simulink model "RTInductionMotorJan27"  (R2020a)
settings: Solver=FixedStepAuto  StartTime=0.0  StopTime=1  RelTol=1e-3
model workspace (MAT data in the model file):
  Fe = 60
  Poles = 2
libraries: powerlib x26, powerlib_meascontrol x4, simulink x1
(part 2 of 2)

== system RTInductionMotorJan27/Motor Model/first test (g results with simscape but without feedback)/Rotor current/Rotor currents ==
  flux_dr : Inport
  flus_qr : Inport  Port=2
  Lr : Inport  Port=3
  Lm : Inport  Port=4
  Add : Sum
  Divide : Product  Inputs=*/
  Divide1 : Product  Inputs=/*
  Lm1 : InportShadow  Port=4
  Product : Product
  Product1 : Product
  Scope : Scope  NumInputPorts=2
  Subtract : Sum  Inputs=-+
  Subtract1 : Sum  Inputs=-+
  i_dr : Outport  VectorParamsAs1DForOutWhenUnconnected=off
  i_qr : Outport  Port=2  VectorParamsAs1DForOutWhenUnconnected=off
  tag scope: i_dr=global, i_qr=global
  wires:
  Divide1/1 -> i_qr/1, Scope/1, [i_qr]  "i_rs"
  Subtract1/1 -> Divide1/2
  flus_qr/1 -> Subtract1/2
  Product1/1 -> Subtract1/1
  [i_qs] -> Product1/2
  Divide/1 -> i_dr/1, Scope/2, [i_dr]  "i_dr"
  Add/1 -> Divide/2, Divide1/1
  Subtract/1 -> Divide/1
  Lm/1 -> Add/2, Product1/1
  Lr/1 -> Add/1
  Product/1 -> Subtract/1
  flux_dr/1 -> Subtract/2
  [i_ds] -> Product/2
  Lm1/1 -> Product/1

== system RTInductionMotorJan27/Motor Model/first test (g results with simscape but without feedback)/Stator current/Stator Flux ==
  Rs (Ohms) : Inport
  w_s : Inport  Port=2
  dq0 : Inport  Port=3
  Demux : Demux  Outputs=3
  Integrator : Integrator
  Integrator1 : Integrator
  Rs (Ohms)1 : InportShadow
  Scope : Scope  NumInputPorts=2
  Subtract : Sum  Inputs=-++
  Subtract1 : Sum  Inputs=-+-
  Terminator : Terminator
  product{,1..3} (4 alike) : Product  Inputs=**
  w_s1 : InportShadow  Port=2
  flux_ds : Outport  VectorParamsAs1DForOutWhenUnconnected=off
  flux_qs : Outport  Port=2  VectorParamsAs1DForOutWhenUnconnected=off
  wires:
  Demux/3 -> Terminator/1
  Demux/2 -> Subtract1/2  "v_qs"
  Demux/1 -> Subtract/2  "v_ds"
  [i_qs] -> product1/2
  product2/1 -> Subtract1/1
  w_s/1 -> product2/2
  product3/1 -> Subtract/3
  w_s1/1 -> product3/1
  Rs (Ohms)1/1 -> product1/1
  Integrator1/1 -> flux_qs/1, Scope/2, product3/2  "flux_qs"
  [i_ds] -> product/1
  product1/1 -> Subtract1/3
  Subtract1/1 -> Integrator1/1
  Integrator/1 -> flux_ds/1, Scope/1, product2/1  "flux_ds"
  Subtract/1 -> Integrator/1
  product/1 -> Subtract/1  "i_ds*R_s"
  Rs (Ohms)/1 -> product/2
  dq0/1 -> Demux/1

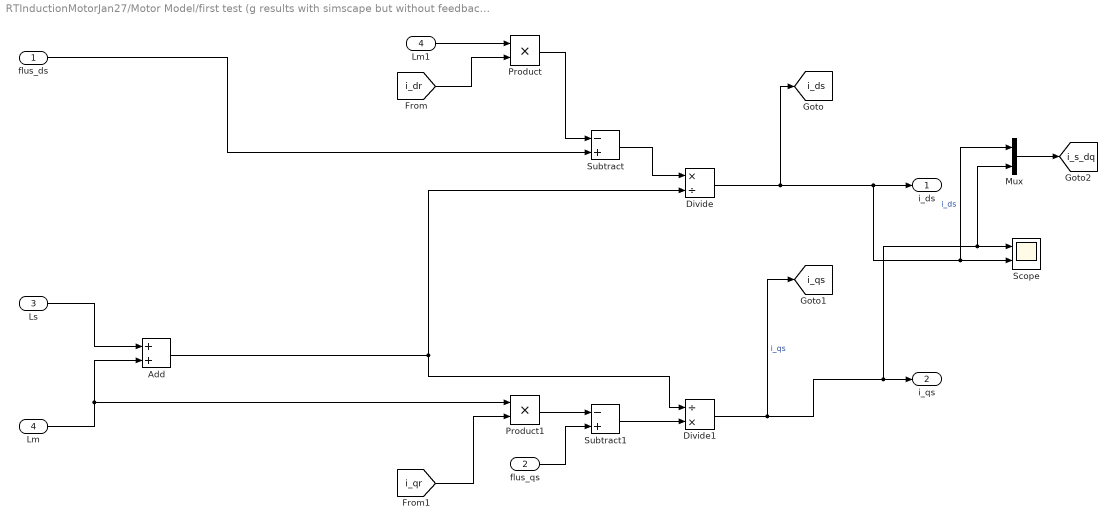
== system RTInductionMotorJan27/Motor Model/first test (g results with simscape but without feedback)/Stator current/Stator currents ==
  flus_ds : Inport
  flus_qs : Inport  Port=2
  Ls : Inport  Port=3
  Lm : Inport  Port=4
  Add : Sum
  Divide : Product  Inputs=*/
  Divide1 : Product  Inputs=/*
  Lm1 : InportShadow  Port=4
  Mux : Mux  Inputs=2
  Product : Product
  Product1 : Product
  Scope : Scope  NumInputPorts=2
  Subtract : Sum  Inputs=-+
  Subtract1 : Sum  Inputs=-+
  i_ds : Outport  VectorParamsAs1DForOutWhenUnconnected=off
  i_qs : Outport  Port=2  VectorParamsAs1DForOutWhenUnconnected=off
  tag scope: i_ds=global, i_qs=global, i_s_dq=global
  wires:
  Mux/1 -> [i_s_dq]
  Divide1/1 -> i_qs/1, Scope/1, Mux/2, [i_qs]  "i_qs"
  Subtract1/1 -> Divide1/2
  flus_qs/1 -> Subtract1/2
  Product1/1 -> Subtract1/1
  [i_qr] -> Product1/2
  Divide/1 -> i_ds/1, Scope/2, Mux/1, [i_ds]  "i_ds"
  Add/1 -> Divide/2, Divide1/1
  Subtract/1 -> Divide/1
  Lm/1 -> Add/2, Product1/1
  Ls/1 -> Add/1
  Product/1 -> Subtract/1
  flus_ds/1 -> Subtract/2
  [i_dr] -> Product/2
  Lm1/1 -> Product/1

== system RTInductionMotorJan27/Motor Model/first test (g results with simscape but without feedback)/dq/Subsystem ==
  P : Inport
  1/60 : Gain  Gain=1/60
  Integrator1 : Integrator
  Math Function : Math  Operator=rem  SignedPower=on  SaturateOnIntegerOverflow=on
  Product : Product
  Product1 : Product
  Two Pi : Constant  Value=2*pi
  w_s (rpm) : Constant  Value=1500
  w_t : Outport  VectorParamsAs1DForOutWhenUnconnected=off
  tag scope: w_s=global
  wires:
  Math Function/1 -> w_t/1
  w_s (rpm)/1 -> Product/1
  P/1 -> Product1/2
  Two Pi/1 -> Product/2, Math Function/2
  1/60/1 -> Integrator1/1, [w_s]  "omega_s"
  Integrator1/1 -> Math Function/1
  Product1/1 -> 1/60/1
  Product/1 -> Product1/1

== system RTInductionMotorJan27/Motor Model/test/Induction Machine/EM Torque ==
  I_s dq : Inport
  I_r dq : Inport  Port=2
  Lm : Inport  Port=3
  P : Inport  Port=4
  Add2 : Sum
  Add3 : Sum
  Add4 : Sum
  Demux2 : Demux  Outputs=2
  Demux3 : Demux  Outputs=2
  Gain1 : Gain  Gain=3/2
  Product{1..3,7..8} (5 alike) : Product
  Scope : Scope
  EM Torque : Outport  VectorParamsAs1DForOutWhenUnconnected=off
  wires:
  Lm/1 -> Product1/2, Product2/2
  I_r dq/1 -> Demux3/1
  Product3/1 -> Gain1/1  "(3 / 2) . p .  (is_q ( Lm ( is_d + ir_d) ) + is_d ( Lm ( is_q + ir_q) ))"
  Demux2/2 -> Product8/2, Add3/1  "Is_q"
  I_s dq/1 -> Demux2/1
  Demux3/1 -> Add2/2  "Ir_d"
  Demux3/2 -> Add3/2  "Ir_q"
  Demux2/1 -> Product7/2, Add2/1  "Is_d"
  Gain1/1 -> Scope/1, EM Torque/1
  Add2/1 -> Product1/1  "is_d + ir_d"
  Add3/1 -> Product2/1  "is_q + ir_q"
  Product2/1 -> Product7/1  "Lm ( is_q + ir_q)"
  Product7/1 -> Add4/2  "is_d ( Lm ( is_q + ir_q) )"
  Product1/1 -> Product8/1  "Lm ( is_d + ir_d)"
  Product8/1 -> Add4/1  "is_q ( Lm ( is_d + ir_d) )"
  Add4/1 -> Product3/1  "is_q ( Lm ( is_d + ir_d) ) + is_d ( Lm ( is_q + ir_q) )"
  P/1 -> Product3/2  "Pole Pairs, P"

== system RTInductionMotorJan27/Motor Model/test/Induction Machine/Fluxes to Currents ==
  Phi_s dq : Inport
  Phi_r dq : Inport  Port=2
  Lm : Inport  Port=3
  Llr : Inport  Port=4
  Lls : Inport  Port=5
  Demux{,1..3} (4 alike) : Demux  Outputs=2
  Mux : Mux  Inputs=2
  Mux1 : Mux  Inputs=2
  Scope : Scope  NumInputPorts=2
  Scope1 : Scope  NumInputPorts=2
  ir_d : Subsystem
  ir_q : Subsystem
  is_d : Subsystem
  is_q : Subsystem
  i_s dq : Outport  VectorParamsAs1DForOutWhenUnconnected=off
  i_r dq : Outport  Port=2  VectorParamsAs1DForOutWhenUnconnected=off
  wires:
  Lls/1 -> is_q/2(Lls), is_d/3(Lls)  "Lls"
  Llr/1 -> ir_d/4(Llr), ir_q/4(Llr)  "Llr"
  Lm/1 -> is_q/1(Lm), is_d/1(Lm), ir_d/3(Lm), ir_q/2(Lm)  "Lm"
  Phi_r dq/1 -> Demux/1
  Phi_s dq/1 -> Demux1/1
  Mux/1 -> i_s dq/1, Demux2/1
  Mux1/1 -> i_r dq/1, Demux3/1
  Demux/2 -> ir_q/1(Phi_r_q)  "Phi_r_q"
  Demux2/2 -> ir_q/3(Is_q)  "is_q"
  ir_q/1(ir_q) -> Scope/2, Mux1/2
  Demux/1 -> ir_d/1(Phi_r_d)  "Phi_r_d"
  Demux2/1 -> ir_d/2(is_d)  "is_d"
  ir_d/1(ir_d) -> Scope/1, Mux1/1
  Demux1/1 -> is_d/2(Phi_s_d)  "Phi_s_d"
  Demux3/1 -> is_d/4(ir_d)  "ir_d"
  is_d/1(is_d) -> Scope1/1, Mux/1
  Demux1/2 -> is_q/3(Phi_s_q)  "Phi_s_q"
  Demux3/2 -> is_q/4(ir_q)  "ir_q"
  is_q/1(is_q) -> Scope1/2, Mux/2

== system RTInductionMotorJan27/Motor Model/test/Induction Machine/Rotor Flux ==
  omega_r : Inport
  omega_s : Inport  Port=2
  I_r dq : Inport  Port=3
  Add1 : Sum  Inputs=+-
  Demux : Demux  Outputs=2
  Integrator : Integrator
  Integrator1 : Integrator
  Mux : Mux  Inputs=2
  Product{,1,3..4} (4 alike) : Product
  Rotor resistance Rr : Constant  Commented=on  Value=0.277
  Rotor resistance Rr1 : Constant  Value=6.085
  Sum : Sum  Inputs=|--
  Sum2 : Sum  Inputs=|+-
  Phi_r dq : Outport  VectorParamsAs1DForOutWhenUnconnected=off
  wires:
  Product3/1 -> Sum2/1  "Phi_r_d . (omega_s - omega_r)"
  omega_r/1 -> Add1/2
  Integrator1/1 -> Product/2, Mux/2  "Phi_r_q"
  Sum2/1 -> Integrator1/1  "(Phi_r_d . (omega_s - omega_r) - (ir_q . Rr)"
  Demux/2 -> Product4/2  "ir_q"
  Product1/1 -> Sum/2  "ir_d . Rr"
  Product4/1 -> Sum2/2  "ir_q . Rr"
  omega_s/1 -> Add1/1
  Product/1 -> Sum/1  "(omega_s - omega_r) . Phi_r_q"
  Add1/1 -> Product/1, Product3/1  "(omega_s - omega_r)"
  Integrator/1 -> Product3/2, Mux/1  "Phi_r_d"
  Sum/1 -> Integrator/1  "- ((omega_s - omega_r) . Phi_r_q) - ir_d . Rr"
  I_r dq/1 -> Demux/1
  Demux/1 -> Product1/2  "ir_d"
  Mux/1 -> Phi_r dq/1
  Rotor resistance Rr1/1 -> Product4/1, Product1/1

== system RTInductionMotorJan27/Motor Model/test/Induction Machine/Rotor Speed ==
  EM Torque (N) : Inport
  Friction (N.m.s) : Inport  Port=2
  Load Torque (N) : Inport  Port=3
  Pole Pairs : Inport  Port=4
  Shaft Innertia (kg . m2) : Inport  Port=5
  Integrator : Integrator
  Product1 : Product  Inputs=*/
  Product2 : Product  Commented=on  Inputs=*/
  Product3 : Product
  Rads-1 --> RPMn : Gain  Commented=on  Gain=60/(2*pi)
  Scope : Scope
  Sum1 : Sum  Inputs=|+-
  Sum2 : Sum  Inputs=|+-
  omega_r_m (RPM) : Outport  VectorParamsAs1DForOutWhenUnconnected=off
  omega_r_e (rads-1) : Outport  Port=2  VectorParamsAs1DForOutWhenUnconnected=off
  wires:
  Product2/1 -> Rads-1 --> RPMn/1
  Product1/1 -> Integrator/1
  Integrator/1 -> Product2/1, Product3/2, Scope/1, omega_r_e (rads-1)/1  "omega_r_e (rads-1)"
  EM Torque (N)/1 -> Sum2/1
  Load Torque (N)/1 -> Sum2/2
  Rads-1 --> RPMn/1 -> omega_r_m (RPM)/1  "omega_r_m (rpm)"
  Sum2/1 -> Sum1/1
  Sum1/1 -> Product1/1  "Net Torque (Nm)"
  Pole Pairs/1 -> Product2/2
  Shaft Innertia (kg . m2)/1 -> Product1/2
  Friction (N.m.s)/1 -> Product3/1  "Frictional Torque (Nm)"
  Product3/1 -> Sum1/2

== system RTInductionMotorJan27/Motor Model/test/Induction Machine/Stator Flux ==
  I_s dq : Inport
  omega_s : Inport  Port=2
  V_s dq0 : Inport  Port=3
  Demux : Demux  Outputs=2
  Demux1 : Demux  Outputs=2
  Integrator1 : Integrator
  Integrator2 : Integrator
  Mux : Mux  Inputs=2
  Product{1,3..5} (4 alike) : Product
  Stator Resistance : Constant  Value=0.183
  Stator Resistance1 : Constant  Value=6.03
  Sum2 : Sum  Inputs=|+-
  Sum3 : Sum  Inputs=|+-
  Sum4 : Sum  Inputs=|+-
  Sum5 : Sum  Inputs=|++
  Phi_s dq : Outport  VectorParamsAs1DForOutWhenUnconnected=off
  wires:
  Sum2/1 -> Sum3/1  "Vs_d - (Is_d . Rs)"
  Demux1/1 -> Product1/1  "I_s d"
  Product3/1 -> Sum3/2  "Phi_s_q . omega_s"
  Sum3/1 -> Integrator1/1  "Vs_d - (Is_d . Rs) + (Phi_s_q . omega_s)"
  Demux/1 -> Sum2/1  "V_s d"
  Demux/2 -> Sum4/1  "V_s q"
  Product4/1 -> Sum4/2
  Integrator1/1 -> Product5/1, Mux/1  "Phi_s_d"
  Demux1/2 -> Product4/1  "I_s q"
  Sum4/1 -> Sum5/1  "Vs_q - (Is_q . Rs)"
  omega_s/1 -> Product5/2, Product3/2
  Product1/1 -> Sum2/2
  Integrator2/1 -> Product3/1, Mux/2  "Phi_s_q"
  Product5/1 -> Sum5/2  "Phi_s_d . omega_s"
  Sum5/1 -> Integrator2/1  "Vs_q - (Is_q . Rs) + (Phi_s_d . omega_s)"
  Mux/1 -> Phi_s dq/1
  I_s dq/1 -> Demux1/1
  V_s dq0/1 -> Demux/1
  Stator Resistance1/1 -> Product4/2, Product1/2

== system RTInductionMotorJan27/Motor Model/test/Induction Machine/abc ==
  Vm : Inport
  Product : Product
  Product1 : Product
  Product2 : Product
  Scope : Scope  NumInputPorts=3
  Sum : Sum  Inputs=--|  InputSameDT=on  SaturateOnIntegerOverflow=on  OutDataTypeStr=Inherit: Same as first input
  V_A : Sin  Frequency=2*pi*60  Phase=pi/2  SampleTime=0
  V_B : Sin  Frequency=2*pi*60  Phase=-pi/6  SampleTime=0
  v_a : Outport  VectorParamsAs1DForOutWhenUnconnected=off
  v_c : Outport  Port=2  VectorParamsAs1DForOutWhenUnconnected=off
  v_b : Outport  Port=3  VectorParamsAs1DForOutWhenUnconnected=off
  wires:
  Vm/1 -> Product2/1, Product1/1, Product/1
  Sum/1 -> Product2/2  "V_C"
  V_A/1 -> Product/2, Sum/2  "A"
  V_B/1 -> Product1/2, Sum/1  "B"
  Product/1 -> Scope/1, v_a/1
  Product1/1 -> Scope/2, v_b/1
  Product2/1 -> v_c/1, Scope/3

== system RTInductionMotorJan27/Motor Model/test/Induction Machine/abc-dq ==
  v_b : Inport
  v_c : Inport  Port=2
  w_s : Inport  Port=3
  v_a : Inport  Port=4
  ABC_to_alpha_beta : Gain  Gain=2/3*[1 -0.5 -0.5;0 0.86667 -0.86667]  Multiplication=Matrix(K*u)  SaturateOnIntegerOverflow=on  OutDataTypeStr=Inherit: Same as input  ParamDataTypeStr=Inherit: Same as input
  Clock : Clock  Commented=on
  Fcn : Fcn  Expr=u(1)*cos(u(3))+u(2)*sin(u(3))
  Fcn1 : Fcn  Expr=-u(1)*sin(u(3))+u(2)*cos(u(3))
  Mux : Mux  Inputs=3
  Mux3 : Mux  Inputs=2
  Mux4 : Mux  Inputs=2
  Mux5 : Mux  Inputs=2
  Product : Product  Commented=on
  Scope1 : Scope
  alpha_beta components : Scope
  t : Clock
  w : Gain  Gain=2*pi*60  SaturateOnIntegerOverflow=on  OutDataTypeStr=Inherit: Same as input  ParamDataTypeStr=Inherit: Same as input
  dq : Outport  VectorParamsAs1DForOutWhenUnconnected=off
  wires:
  Mux/1 -> ABC_to_alpha_beta/1  "ABC"
  ABC_to_alpha_beta/1 -> Mux4/1, Mux3/1, alpha_beta components/1  "ab"
  v_a/1 -> Mux/1
  v_b/1 -> Mux/2
  v_c/1 -> Mux/3
  Clock/1 -> Product/1
  w_s/1 -> Product/2
  Fcn1/1 -> Mux5/2
  Fcn/1 -> Mux5/1
  w/1 -> Mux3/2, Mux4/2
  Mux3/1 -> Fcn/1
  Mux5/1 -> Scope1/1, dq/1
  Mux4/1 -> Fcn1/1
  t/1 -> w/1

== system RTInductionMotorJan27/Motor Model/test/Induction Machine/Fluxes to Currents/ir_d ==
  Phi_r_d : Inport
  is_d : Inport  Port=2
  Lm : Inport  Port=3
  Llr : Inport  Port=4
  Add1 : Sum  Inputs=+-
  Add3 : Sum
  Product1 : Product
  Product3 : Product  Inputs=*/
  ir_d : Outport  VectorParamsAs1DForOutWhenUnconnected=off
  wires:
  is_d/1 -> Product1/1
  Add1/1 -> Product3/1  "Phi_r_d - (is_d . Lm)"
  Add3/1 -> Product3/2  "Lm + Llr"
  Product1/1 -> Add1/2  "is_d . Lm"
  Phi_r_d/1 -> Add1/1
  Lm/1 -> Add3/1, Product1/2
  Llr/1 -> Add3/2
  Product3/1 -> ir_d/1  "(Phi_r_d - (is_d . Lm)) / (Lm+Llr)"

== system RTInductionMotorJan27/Motor Model/test/Induction Machine/Fluxes to Currents/ir_q ==
  Phi_r_q : Inport
  Lm : Inport  Port=2
  Is_q : Inport  Port=3
  Llr : Inport  Port=4
  Add7 : Sum  Inputs=+-
  Add8 : Sum
  Product7 : Product
  Product8 : Product  Inputs=*/
  ir_q : Outport  VectorParamsAs1DForOutWhenUnconnected=off
  wires:
  Lm/1 -> Product7/2, Add8/1
  Llr/1 -> Add8/2
  Product8/1 -> ir_q/1  "(Phi_r_q - (is_q . Lm)) / (Lm + Llr)"
  Product7/1 -> Add7/2  "is_q . Lm"
  Phi_r_q/1 -> Add7/1
  Add7/1 -> Product8/1  "Phi_r_q - (is_q . Lm)"
  Add8/1 -> Product8/2  "Lm+Llr"
  Is_q/1 -> Product7/1

== system RTInductionMotorJan27/Motor Model/test/Induction Machine/Fluxes to Currents/is_d ==
  Lm : Inport
  Phi_s_d : Inport  Port=2
  Lls : Inport  Port=3
  ir_d : Inport  Port=4
  Add2 : Sum  Inputs=+-
  Add4 : Sum
  Product2 : Product
  Product4 : Product  Inputs=*/
  is_d : Outport  VectorParamsAs1DForOutWhenUnconnected=off
  wires:
  Product4/1 -> is_d/1  "(Phi_s_d - (ir_d . Lm)) / (Lm + Lls)"
  Lm/1 -> Product2/2, Add4/1
  Lls/1 -> Add4/2
  Product2/1 -> Add2/2  "ir_d . Lm"
  Phi_s_d/1 -> Add2/1
  Add4/1 -> Product4/2  "Lm + Lls"
  ir_d/1 -> Product2/1
  Add2/1 -> Product4/1  "Phi_s_d - (ir_d . Lm)"

== system RTInductionMotorJan27/Motor Model/test/Induction Machine/Fluxes to Currents/is_q ==
  Lm : Inport
  Lls : Inport  Port=2
  Phi_s_q : Inport  Port=3
  ir_q : Inport  Port=4
  Add5 : Sum  Inputs=+-
  Add6 : Sum
  Product5 : Product
  Product6 : Product  Inputs=*/
  is_q : Outport  VectorParamsAs1DForOutWhenUnconnected=off
  wires:
  Lls/1 -> Add6/2
  Lm/1 -> Product5/2, Add6/1
  ir_q/1 -> Product5/1
  Add6/1 -> Product6/2
  Add5/1 -> Product6/1
  Phi_s_q/1 -> Add5/1
  Product6/1 -> is_q/1
  Product5/1 -> Add5/2
